simulink model "simple_example"  (R2016a)
settings: Solver=ode45  StartTime=0.0  StopTime=500  RelTol=1e-3
InitFcn:
  | param
undefined symbols (not defined in the file or in its folder): ctrl, P
settings Model: Creator=beard  LastModifiedBy=beard
settings DataIOCC: LimitDataPoints=on  SaveFormat=Array
settings DebuggingCC: UnderspecifiedInitializationDetection=Classic  MergeDetectMultiDrivingBlocksExec=none  SolverPrmCheckMsg=warning  StateNameClashWarn=warning
settings HardwareCC: ProdBitPerPointer=32  ProdLargestAtomicFloat=None  ProdIntDivRoundTo=Undefined  ProdEndianess=Unspecified  ProdWordSize=32  ProdHWDeviceType=32-bit Generic
settings ModelReferenceCC: PropagateSignalLabelsOutOfModel=off
settings ConfigComp: CovModelRefEnable=Off

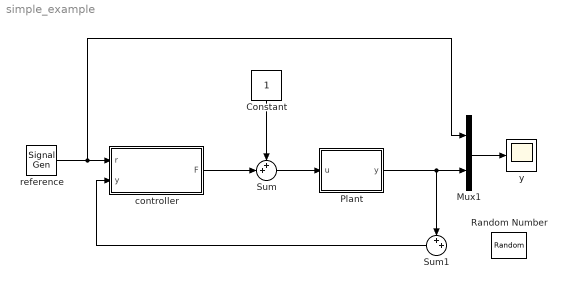
== system simple_example ==
  Constant : Constant
  Mux1 : Mux  Inputs=2
  Plant : Subsystem
  Random Number : RandomNumber  Variance=.01^2  SampleTime=0.1
  Sum : Sum  Inputs=++|
  Sum1 : Sum  Inputs=++|
  controller : Subsystem
  reference : SignalGenerator  WaveForm=square  Frequency=0.01
  y : Scope
  wires:
  controller/1(F) -> Sum/2
  Plant/1(y) -> Sum1/1, Mux1/2
  Sum/1 -> Plant/1(u)
  Mux1/1 -> y/1
  reference/1 -> Mux1/1, controller/1(r)
  Sum1/1 -> controller/2(y)
  Constant/1 -> Sum/1

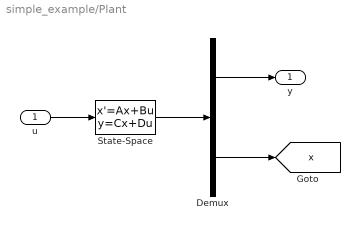
== system simple_example/Plant ==
  u : Inport
  Demux : Demux  Outputs=[1;2]
  State-Space : StateSpace  A=P.A+0.0*randn(2,2)  B=P.B  C=[P.C; eye(2)]  D=[P.D; 0; 0]  X0=[0;0]
  y : Outport
  tag scope: x=global
  wires:
  u/1 -> State-Space/1
  State-Space/1 -> Demux/1
  Demux/1 -> y/1
  Demux/2 -> [x]

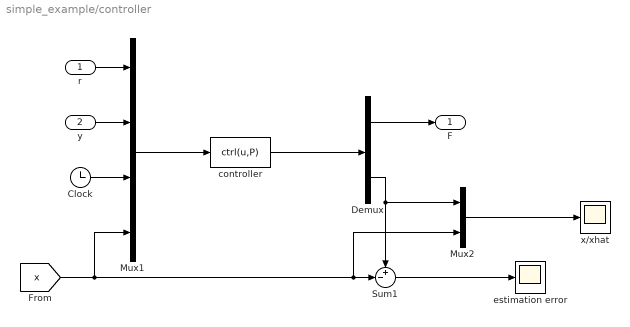
== system simple_example/controller ==
  r : Inport
  y : Inport  Port=2
  Clock : Clock
  Demux : Demux  Outputs=[1;2]
  Mux1 : Mux
  Mux2 : Mux  Inputs=2
  Sum1 : Sum  Inputs=+-|
  controller : MATLABFcn  MATLABFcn=ctrl(u,P)  OutputDimensions=1+2  SampleTime=P.Ts
  estimation error : Scope
  x/xhat : Scope
  F : Outport
  wires:
  Clock/1 -> Mux1/3
  y/1 -> Mux1/2
  r/1 -> Mux1/1
  Mux1/1 -> controller/1
  Demux/1 -> F/1
  controller/1 -> Demux/1
  [x] -> Mux1/4, Mux2/2, Sum1/2
  Demux/2 -> Mux2/1, Sum1/1
  Sum1/1 -> estimation error/1
  Mux2/1 -> x/xhat/1
